simulink model "OOK"  (Simulink 7.2)
settings: Solver=ode45  StartTime=0.0  StopTime=100  RelTol=1e-3
libraries: commrandsrc2 x1, dsparch4 x1
settings Model: Creator=usuario  LastModifiedBy=USUARIO
settings OptimizationCC: InitFltsAndDblsToZero=on
settings DebuggingCC: SaveWithParameterizedLinksMsg=none  SignalResolutionControl=TryResolveAllWithWarning  MultiTaskDSMMsg=warning  MultiTaskCondExecSysMsg=none
settings RTWCC: IncludeERTFirstTime=on
settings GRTTargetCC: TargetFcnLib=ansi_tfl_tmw.mat

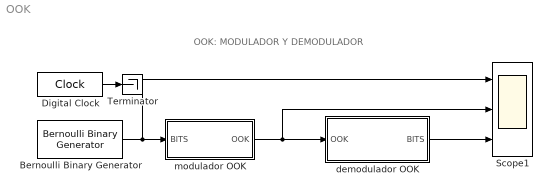
== system OOK ==
  note: OOK: MODULADOR Y DEMODULADOR
  Bernoulli Binary Generator : commrandsrc2/Bernoulli Binary Generator  DialogController=commDDGCreate  DialogControllerArgs=DataTag0  SystemSampleTime=-1  P=0.5  seed=51  Ts=5  frameBased=off  sampPerFrame=1  orient=off  outDataType=double
  Digital Clock : DigitalClock  SampleTime=0.001
  Scope1 : Scope  NumInputPorts=3
      settings: YMin=-5~-5~-5  YMax=5~5~5  SaveName=ScopeData3
  Terminator : Terminator
  demodulador OOK : Subsystem
  modulador OOK : Subsystem
  wires:
  Bernoulli Binary Generator/1 -> modulador OOK/1(BITS), Scope1/1
  modulador OOK/1(OOK) -> demodulador OOK/1(OOK), Scope1/2
  demodulador OOK/1(BITS) -> Scope1/3
  Digital Clock/1 -> Terminator/1

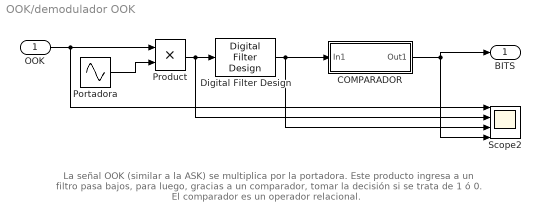
== system OOK/demodulador OOK ==
  note: La señal OOK (similar a la ASK) se multiplica por la portadora.
      | Este producto ingresa a un filtro
      | pasa bajos, para luego, gracias a un
      | comparador, tomar la decisión si se trata de
      | 1 ó 0. El comparador es un operador relacional.
  OOK : Inport  OutDataType=sfix(16)  OutScaling=2^0
  COMPARADOR : Subsystem
  Digital Filter Design : dsparch4/Digital Filter Design  SystemSampleTime=-1  mwdsp_browser_bugfix_var=off
  Portadora : Sin  SineType=Sample based  Frequency=2*10*pi  Samples=50  SampleTime=1/20
  Product : Product  OutDataType=sfix(16)  OutScaling=2^0  RndMeth=Zero
  Scope2 : Scope  NumInputPorts=4
      settings: YMin=-2~-3~-3~-5  YMax=2~3~3~5
  BITS : Outport  OutDataType=sfix(16)  OutScaling=2^0
  wires:
  OOK/1 -> Scope2/1, Product/1
  Portadora/1 -> Product/2
  Product/1 -> Digital Filter Design/1, Scope2/2
  Digital Filter Design/1 -> Scope2/3, COMPARADOR/1(In1)
  COMPARADOR/1(Out1) -> Scope2/4, BITS/1

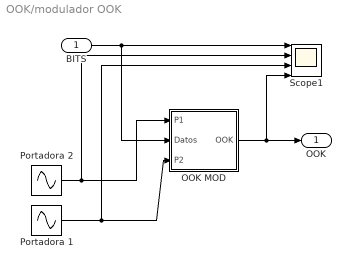
== system OOK/modulador OOK ==
  BITS : Inport  OutDataType=sfix(16)  OutScaling=2^0
  OOK MOD : Subsystem
  Portadora 1 : Sin  SineType=Sample based  Amplitude=0  Frequency=2*10*pi  Phase=-pi  Samples=50  SampleTime=1/20
  Portadora 2 : Sin  SineType=Sample based  Amplitude=2  Frequency=2*10*pi  Samples=50  SampleTime=1/20
  Scope1 : Scope  NumInputPorts=4
      settings: YMin=-2~-3~-3~-3  YMax=2~3~3~3
  OOK : Outport  OutDataType=sfix(16)  OutScaling=2^0
  wires:
  BITS/1 -> Scope1/1, OOK MOD/2(Datos)
  Portadora 2/1 -> Scope1/2, OOK MOD/1(P1)
  Portadora 1/1 -> Scope1/3, OOK MOD/3(P2)
  OOK MOD/1(OOK) -> OOK/1, Scope1/4

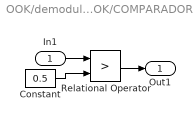
== system OOK/demodulador OOK/COMPARADOR ==
  In1 : Inport  OutDataType=sfix(16)  OutScaling=2^0
  Constant : Constant  Value=0.5  OutDataType=sfix(16)  OutScaling=2^0
  Relational Operator : RelationalOperator  Operator=>  LogicOutDataTypeMode=boolean  OutDataTypeStr=boolean
  Out1 : Outport  OutDataType=sfix(16)  OutScaling=2^0
  wires:
  Constant/1 -> Relational Operator/2
  In1/1 -> Relational Operator/1
  Relational Operator/1 -> Out1/1

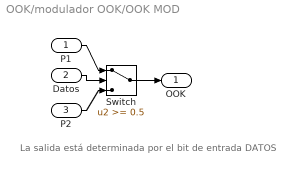
== system OOK/modulador OOK/OOK MOD ==
  note: La salida está
      | determinada por
      | el bit de entrada DATOS
  P1 : Inport  OutDataType=sfix(16)  OutScaling=2^0
  Datos : Inport  Port=2  OutDataType=sfix(16)  OutScaling=2^0
  P2 : Inport  Port=3  OutDataType=sfix(16)  OutScaling=2^0
  Switch : Switch  Threshold=0.5
  OOK : Outport  OutDataType=sfix(16)  OutScaling=2^0
  wires:
  P1/1 -> Switch/1
  Datos/1 -> Switch/2
  Switch/1 -> OOK/1
  P2/1 -> Switch/3
